simulink model "FusionMODEL_version1"  (R2018a)
settings: Solver=FixedStepAuto  StartTime=0.0  StopTime=SimulationTime  FixedStep=SamplingTime  RelTol=1e-3
undefined symbols (not defined in the file or in its folder): ACTIVATE_CAM, ACTIVATE_RAD, CAM1_detTimeStamp, CAM1_MeasNoise, CAM1_objClassID, CAM1_PX, CAM1_PY, CAM1_VX, CAM1_VY, CAM2_detTimeStamp, CAM2_MeasNoise, CAM2_objClassID, CAM2_PX, CAM2_PY, CAM2_VX, CAM2_VY, CAM3_detTimeStamp, CAM3_MeasNoise, CAM3_objClassID, CAM3_PX, CAM3_PY, CAM3_VX, CAM3_VY, CAM4_detTimeStamp, CAM4_MeasNoise, CAM4_objClassID, CAM4_PX, CAM4_PY, CAM4_VX, CAM4_VY, CAM5_detTimeStamp, CAM5_MeasNoise, CAM5_objClassID, CAM5_PX, CAM5_PY, CAM5_VX, CAM5_VY, CAM6_detTimeStamp, CAM6_MeasNoise, CAM6_objClassID, CAM6_PX, CAM6_PY, CAM6_VX, CAM6_VY, CAM7_detTimeStamp, CAM7_MeasNoise, CAM7_objClassID, CAM7_PX, CAM7_PY, CAM7_VX, CAM7_VY, CAM8_detTimeStamp, CAM8_MeasNoise, CAM8_objClassID, CAM8_PX, CAM8_PY, CAM8_VX, CAM8_VY, CAM_nMeas, CAM_TYPE ... (+151)
libraries: simulink_extras x2
(part 3 of 6)

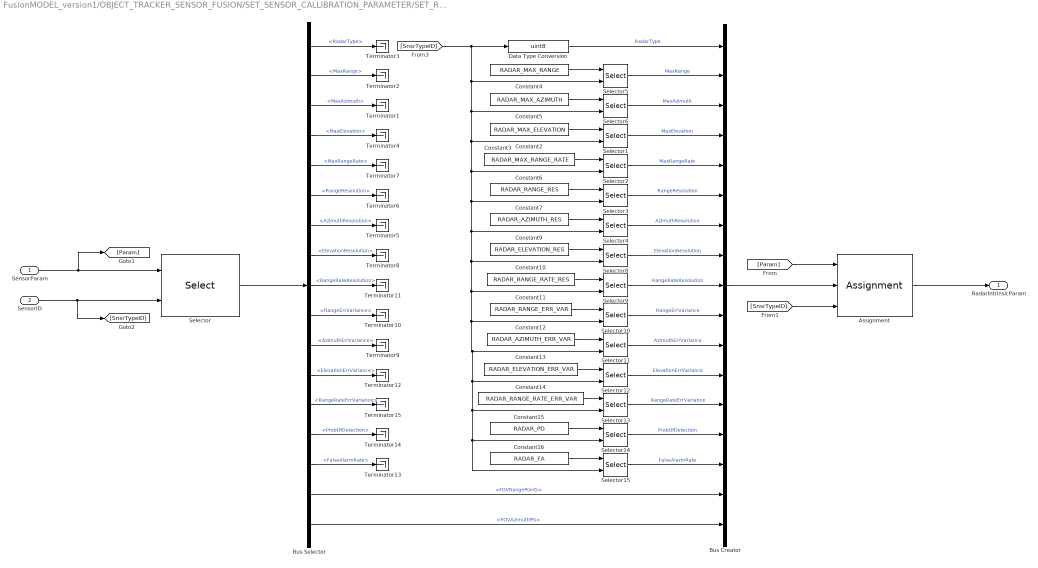
== system FusionMODEL_version1/OBJECT_TRACKER_SENSOR_FUSION/SET_SENSOR_CALLIBRATION_PARAMETER/SET_RADAR_SENSOR_PARAM/SET_RADAR_INTRINSIC_PARAM/SET_RADAR_INTRINSIC_PARAM ==
  SensorParam : Inport
  SensorID : Inport  Port=2
  Assignment : Assignment  DiagnosticForDimensions=Warning  IndexOptions=Index vector (port)  Indices=1  OutputSizes=1
  Bus Creator : BusCreator  Inputs=17  OutDataTypeStr=Bus: RadarIntrinsicParam  NonVirtualBus=on
  Bus Selector : BusSelector  OutputSignals=RadarType,MaxRange,MaxAzimuth,MaxElevation,MaxRangeRate,RangeResolution,AzimuthResolution,ElevationResolution,RangeRateResolution,RangeErrVariance,AzimuthErrVariance,ElevationErrVariance,RangeRateErrVariance,ProbOfDetection,FalseAlarmRate,FOVRangePoints,FOVAzimuthPts
  Constant10 : Constant  Value=RADAR_RANGE_RATE_RES
  Constant11 : Constant  Value=RADAR_RANGE_ERR_VAR
  Constant12 : Constant  Value=RADAR_AZIMUTH_ERR_VAR
  Constant13 : Constant  Value=RADAR_ELEVATION_ERR_VAR
  Constant14 : Constant  Value=RADAR_RANGE_RATE_ERR_VAR
  Constant15 : Constant  Value=RADAR_PD
  Constant16 : Constant  Value=RADAR_FA
  Constant2 : Constant  Value=RADAR_MAX_ELEVATION
  Constant3 : Constant  Value=RADAR_MAX_RANGE_RATE
  Constant4 : Constant  Value=RADAR_MAX_RANGE
  Constant5 : Constant  Value=RADAR_MAX_AZIMUTH
  Constant6 : Constant  Value=RADAR_RANGE_RES
  Constant7 : Constant  Value=RADAR_AZIMUTH_RES
  Constant9 : Constant  Value=RADAR_ELEVATION_RES
  Data Type Conversion : DataTypeConversion  OutDataTypeStr=uint8
  Selector{,1..6,8..15} (15 alike) : Selector  InputPortWidth=nRadarTypes  IndexOptions=Index vector (port)  Indices=[1 3]  OutputSizes=1
  Terminator{1..15} (15 alike) : Terminator
  RadarIntrinsicParam : Outport
  wires:
  Assignment/1 -> RadarIntrinsicParam/1
  SensorParam/1 -> [Param], Selector/1
  Selector/1 -> Bus Selector/1
  Bus Creator/1 -> Assignment/2
  SensorID/1 -> [SnsrTypeID], Selector/2
  [Param] -> Assignment/1
  [SnsrTypeID] -> Assignment/3
  Bus Selector/17 -> Bus Creator/17  "<FOVAzimuthPts>"
  Bus Selector/16 -> Bus Creator/16  "<FOVRangePoints>"
  Constant5/1 -> Selector6/1
  Constant4/1 -> Selector5/1
  Bus Selector/3 -> Terminator1/1  "<MaxAzimuth>"
  Bus Selector/2 -> Terminator2/1  "<MaxRange>"
  Bus Selector/1 -> Terminator3/1  "<RadarType>"
  Selector6/1 -> Bus Creator/3  "MaxAzimuth"
  Selector5/1 -> Bus Creator/2  "MaxRange"
  [SnsrTypeID] -> Selector14/2, Selector15/2, Selector13/2, Selector12/2, Selector11/2, Selector10/2, Selector9/2, Selector8/2, Selector4/2, Selector3/2, Selector2/2, Selector1/2, Selector6/2, Selector5/2, Data Type Conversion/1
  Selector1/1 -> Bus Creator/4  "MaxElevation"
  Selector2/1 -> Bus Creator/5  "MaxRangeRate"
  Selector3/1 -> Bus Creator/6  "RangeResolution"
  Selector4/1 -> Bus Creator/7  "AzimuthResolution"
  Selector8/1 -> Bus Creator/8  "ElevationResolution"
  Constant2/1 -> Selector1/1
  Constant3/1 -> Selector2/1
  Constant6/1 -> Selector3/1
  Constant7/1 -> Selector4/1
  Constant9/1 -> Selector8/1
  Selector9/1 -> Bus Creator/9  "RangeRateResolution"
  Selector10/1 -> Bus Creator/10  "RangeErrVariance"
  Selector11/1 -> Bus Creator/11  "AzimuthErrVariance"
  Selector12/1 -> Bus Creator/12  "ElevationErrVariance"
  Selector13/1 -> Bus Creator/13  "RangeRateErrVariance"
  Selector14/1 -> Bus Creator/14  "ProbOfDetection"
  Selector15/1 -> Bus Creator/15  "FalseAlarmRate"
  Constant10/1 -> Selector9/1
  Constant11/1 -> Selector10/1
  Constant12/1 -> Selector11/1
  Constant13/1 -> Selector12/1
  Constant14/1 -> Selector13/1
  Constant15/1 -> Selector14/1
  Constant16/1 -> Selector15/1
  Bus Selector/4 -> Terminator4/1  "<MaxElevation>"
  Bus Selector/7 -> Terminator5/1  "<AzimuthResolution>"
  Bus Selector/6 -> Terminator6/1  "<RangeResolution>"
  Bus Selector/8 -> Terminator8/1  "<ElevationResolution>"
  Bus Selector/5 -> Terminator7/1  "<MaxRangeRate>"
  Bus Selector/11 -> Terminator9/1  "<AzimuthErrVariance>"
  Bus Selector/14 -> Terminator14/1  "<ProbOfDetection>"
  Bus Selector/10 -> Terminator10/1  "<RangeErrVariance>"
  Bus Selector/13 -> Terminator15/1  "<RangeRateErrVariance>"
  Bus Selector/12 -> Terminator12/1  "<ElevationErrVariance>"
  Bus Selector/15 -> Terminator13/1  "<FalseAlarmRate>"
  Bus Selector/9 -> Terminator11/1  "<RangeRateResolution>"
  Data Type Conversion/1 -> Bus Creator/1  "RadarType"

== system FusionMODEL_version1/OBJECT_TRACKER_SENSOR_FUSION/SPATIAL_ALLIGNMENT/CAMERA_MEASUREMENTS_SPATIAL_ALLIGNMENT/For Iterator Subsystem/For Iterator Subsystem ==
  CameraCalibration : Inport
  nMeas : Inport  Port=2
  CameraCAN : Inport  Port=3
  CoordinateTransformation1 : Subsystem  TreatAsAtomicUnit=on
  For Iterator : ForIterator  ResetStates=reset  IterationSource=external
  SetMeasurement : Subsystem  Commented=on
  SetMeasurement1 : Subsystem
  Subsystem : Subsystem
  nValidMeas : Outport
  CameraMeasUpd : Outport  Port=2
  CameraMeasNoiseCovUpd : Outport  Port=3
  CameraMeasRefUpd : Outport  Port=4
  wires:
  nMeas/1 -> For Iterator/1
  CameraCalibration/1 -> CoordinateTransformation1/2(SensorParam)
  CameraCAN/1 -> Subsystem/1(measCAN)
  For Iterator/1 -> [CamCANidx], Subsystem/2(measIdx)
  Subsystem/4(meas_i) -> SetMeasurement1/4(CameraMeasCAN), CoordinateTransformation1/1(meas)
  Subsystem/3(nValidMeasCnt) -> nValidMeas/1
  Subsystem/2(measID) -> [measID]
  Subsystem/1(isValid) -> CoordinateTransformation1/Action
  CoordinateTransformation1/1(measUpd) -> SetMeasurement1/1(measTransformed)
  [measID] -> SetMeasurement1/2(measID)
  [CamCANidx] -> SetMeasurement1/3(CamCANidx)
  SetMeasurement1/1(CameraCTSMatUpd) -> CameraMeasUpd/1, SetMeasurement1/5(CameraMeasCTSMat)
  SetMeasurement1/2(CameraCTSNoiseCovMatUpd) -> CameraMeasNoiseCovUpd/1, SetMeasurement1/6(CameraMeasCTSNoiseMat)
  SetMeasurement1/3(CameraCTSRefUpd) -> CameraMeasRefUpd/1, SetMeasurement1/7(CameraMeasCTSRef)

== system FusionMODEL_version1/OBJECT_TRACKER_SENSOR_FUSION/SPATIAL_ALLIGNMENT/CAMERA_MEASUREMENTS_SPATIAL_ALLIGNMENT/For Iterator Subsystem/InformationExtraction ==
  CameraCallibration : Inport
  CameraID : Inport  Port=2
  C1 : Inport  Port=3
  C2 : Inport  Port=4
  C3 : Inport  Port=5
  C4 : Inport  Port=6
  C5 : Inport  Port=7
  C6 : Inport  Port=8
  C7 : Inport  Port=9
  C8 : Inport  Port=10
  StartingIndexes : Inport  Port=11
  Bus Selector : BusSelector  OutputSignals=nMeas
  Multiport Switch : MultiPortSwitch  Inputs=8
  Reshape : Reshape  OutputDimensionality=Row vector (2-D)
  Selector : Selector  NumberOfDimensions=2  InputPortWidth=3  IndexOptions=Select all,Index vector (port)  Indices=[1 3],1  OutputSizes=1,1
  Selector1 : Selector  NumberOfDimensions=2  InputPortWidth=3  IndexOptions=Select all,Index vector (port)  Indices=[1 3],1  OutputSizes=1,1
  CameraCalib : Outport
  nCameraMeas : Outport  Port=2
  CameraCANBus : Outport  Port=3
  MeasStartingIdx : Outport  Port=4
  wires:
  CameraCallibration/1 -> Selector/1
  Selector/1 -> CameraCalib/1, Bus Selector/1
  Bus Selector/1 -> nCameraMeas/1  "<nMeas>"
  CameraID/1 -> Selector1/2, Multiport Switch/1, Selector/2
  C1/1 -> Multiport Switch/2
  C2/1 -> Multiport Switch/3
  C3/1 -> Multiport Switch/4
  C4/1 -> Multiport Switch/5
  C5/1 -> Multiport Switch/6
  C6/1 -> Multiport Switch/7
  Multiport Switch/1 -> Reshape/1
  Selector1/1 -> MeasStartingIdx/1
  StartingIndexes/1 -> Selector1/1
  Reshape/1 -> CameraCANBus/1
  C7/1 -> Multiport Switch/8
  C8/1 -> Multiport Switch/9

== system FusionMODEL_version1/OBJECT_TRACKER_SENSOR_FUSION/SPATIAL_ALLIGNMENT/CAMERA_MEASUREMENTS_SPATIAL_ALLIGNMENT/For Iterator Subsystem/Subsystem ==
  nValidMeasVectorIn : Inport
  SnsrIndex : Inport  Port=2
  nValidMeas : Inport  Port=3
  CameraCTSMeas : Inport  Port=4
  CameraCTSNoiseCOV : Inport  Port=5
  CameraCTSRef : Inport  Port=6
  StartIdx : Inport  Port=7
  CTSMeasAllSensors : Inport  Port=8
  CTSNoiseCOV : Inport  Port=9
  CTSRef : Inport  Port=10
  Add : Sum
  Assignment : Assignment  NumberOfDimensions=2  DiagnosticForDimensions=Warning  IndexOptions=Assign all,Index vector (port)  Indices=1,1  OutputSizes=1,1
  Assignment1 : Assignment  NumberOfDimensions=2  DiagnosticForDimensions=Warning  IndexOptions=Assign all,Starting index (port)  Indices=1,1  OutputSizes=1,1
  Assignment2 : Assignment  NumberOfDimensions=3  DiagnosticForDimensions=Warning  IndexOptions=Assign all,Assign all,Starting index (port)  Indices=1,1,1  OutputSizes=1,1,1
  Assignment3 : Assignment  NumberOfDimensions=2  DiagnosticForDimensions=Warning  IndexOptions=Assign all,Starting index (port)  Indices=1,1  OutputSizes=1,1
  Constant2 : Constant  Value=int32(1)
  Data Type Conversion : DataTypeConversion  OutDataTypeStr=uint16
  Reshape : Reshape  OutputDimensionality=Row vector (2-D)
  Unit Delay : UnitDelay  InitialCondition=single(zeros(2, 1600))  SampleTime=-1
  Unit Delay1 : UnitDelay  InitialCondition=uint16(zeros(1,8))  SampleTime=-1
  Unit Delay2 : UnitDelay  InitialCondition=single(zeros(2, 2, 1600))  SampleTime=-1
  Unit Delay3 : UnitDelay  InitialCondition=uint16(zeros(2, 1600))  SampleTime=-1
  nValidMeasVector : Outport
  CTSMat : Outport  Port=2
  CTSMatNoiseCOV : Outport  Port=3
  CTSMatRef : Outport  Port=4
  wires:
  nValidMeas/1 -> Data Type Conversion/1
  SnsrIndex/1 -> Assignment/3
  Assignment/1 -> nValidMeasVector/1
  Unit Delay1/1 -> Reshape/1
  CTSMeasAllSensors/1 -> Unit Delay/1
  CameraCTSMeas/1 -> Assignment1/2
  Assignment1/1 -> CTSMat/1
  StartIdx/1 -> Add/1
  Constant2/1 -> Add/2
  Data Type Conversion/1 -> Assignment/2
  Reshape/1 -> Assignment/1
  nValidMeasVectorIn/1 -> Unit Delay1/1
  Unit Delay/1 -> Assignment1/1
  Unit Delay2/1 -> Assignment2/1
  CameraCTSNoiseCOV/1 -> Assignment2/2
  Add/1 -> Assignment3/3, Assignment2/3, Assignment1/3
  Assignment2/1 -> CTSMatNoiseCOV/1
  Assignment3/1 -> CTSMatRef/1
  CameraCTSRef/1 -> Assignment3/2
  Unit Delay3/1 -> Assignment3/1
  CTSNoiseCOV/1 -> Unit Delay2/1
  CTSRef/1 -> Unit Delay3/1

== system FusionMODEL_version1/OBJECT_TRACKER_SENSOR_FUSION/SPATIAL_ALLIGNMENT/CAMERA_MEASUREMENTS_SPATIAL_ALLIGNMENT/StartingIndexes1/CallibrationInfoExtractor ==
  SnsrCallib : Inport
  Bus Selector{,1..7} (8 alike) : BusSelector  OutputSignals=nMeas
  Selector : Selector  InputPortWidth=nCameras  IndexOptions=Index vector (dialog)  Indices=1  OutputSizes=1
  Selector1 : Selector  InputPortWidth=nCameras  IndexOptions=Index vector (dialog)  Indices=2  OutputSizes=1
  Selector2 : Selector  InputPortWidth=nCameras  IndexOptions=Index vector (dialog)  Indices=3  OutputSizes=1
  Selector3 : Selector  InputPortWidth=nCameras  IndexOptions=Index vector (dialog)  Indices=4  OutputSizes=1
  Selector4 : Selector  InputPortWidth=nCameras  IndexOptions=Index vector (dialog)  Indices=5  OutputSizes=1
  Selector5 : Selector  InputPortWidth=nCameras  IndexOptions=Index vector (dialog)  Indices=7  OutputSizes=1
  Selector6 : Selector  InputPortWidth=nCameras  IndexOptions=Index vector (dialog)  Indices=6  OutputSizes=1
  Selector7 : Selector  InputPortWidth=nCameras  IndexOptions=Index vector (dialog)  Indices=8  OutputSizes=1
  Terminator : Terminator
  C1nMeas : Outport
  C2nMeas : Outport  Port=2
  C3nMeas : Outport  Port=3
  C4nMeas : Outport  Port=4
  C5nMeas : Outport  Port=5
  C6nMeas : Outport  Port=6
  C7nMeas : Outport  Port=7
  wires:
  Bus Selector4/1 -> C5nMeas/1  "<nMeas>"
  Selector4/1 -> Bus Selector4/1
  Bus Selector1/1 -> C2nMeas/1  "<nMeas>"
  Selector1/1 -> Bus Selector1/1
  Selector2/1 -> Bus Selector2/1
  Bus Selector2/1 -> C3nMeas/1  "<nMeas>"
  Selector6/1 -> Bus Selector5/1
  Selector/1 -> Bus Selector/1
  Selector3/1 -> Bus Selector3/1
  Bus Selector3/1 -> C4nMeas/1  "<nMeas>"
  Bus Selector/1 -> C1nMeas/1  "<nMeas>"
  Bus Selector5/1 -> C6nMeas/1  "<nMeas>"
  Selector5/1 -> Bus Selector6/1
  Bus Selector6/1 -> C7nMeas/1  "<nMeas>"
  Bus Selector7/1 -> Terminator/1  "<nMeas>"
  Selector7/1 -> Bus Selector7/1
  SnsrCallib/1 -> Selector7/1, Selector5/1, Selector6/1, Selector4/1, Selector3/1, Selector2/1, Selector1/1, Selector/1

== system FusionMODEL_version1/OBJECT_TRACKER_SENSOR_FUSION/SPATIAL_ALLIGNMENT/CAMERA_MEASUREMENTS_SPATIAL_ALLIGNMENT/StartingIndexes1/Subsystem ==
  C1nMeas : Inport
  C2nMeas : Inport  Port=2
  C3nMeas : Inport  Port=3
  C4nMeas : Inport  Port=4
  C5nMeas : Inport  Port=5
  C6nMeas : Inport  Port=6
  C7nMeas : Inport  Port=7
  Add{,1..5} (6 alike) : Sum
  Constant : Constant  Value=int32(0)
  Data Type Conversion{,1..6} (7 alike) : DataTypeConversion  OutDataTypeStr=int32
  Mux : Mux  Inputs=8
  Reshape : Reshape  OutputDimensionality=Row vector (2-D)
  StartingIndexes : Outport
  wires:
  [C1] -> Mux/1
  Add/1 -> [C3], Add1/1
  Add1/1 -> [C4], Add2/1
  Data Type Conversion3/1 -> Add2/2
  [C4] -> Mux/4
  [C2] -> Mux/2
  Add3/1 -> Add4/1, [C6]
  Constant/1 -> [C1]
  Add2/1 -> [C5], Add3/1
  [C5] -> Mux/5
  [C6] -> Mux/6
  C5nMeas/1 -> Data Type Conversion4/1
  Data Type Conversion/1 -> [C2], Add/1
  [C3] -> Mux/3
  Data Type Conversion1/1 -> Add/2
  Data Type Conversion2/1 -> Add1/2
  Data Type Conversion4/1 -> Add3/2
  C3nMeas/1 -> Data Type Conversion2/1
  C1nMeas/1 -> Data Type Conversion/1
  C2nMeas/1 -> Data Type Conversion1/1
  Mux/1 -> Reshape/1
  C4nMeas/1 -> Data Type Conversion3/1
  Reshape/1 -> StartingIndexes/1
  C6nMeas/1 -> Data Type Conversion5/1
  C7nMeas/1 -> Data Type Conversion6/1
  Data Type Conversion5/1 -> Add4/2
  Data Type Conversion6/1 -> Add5/2
  Add4/1 -> [C7], Add5/1
  Add5/1 -> [C8]
  [C7] -> Mux/7
  [C8] -> Mux/8

== system FusionMODEL_version1/OBJECT_TRACKER_SENSOR_FUSION/SPATIAL_ALLIGNMENT/RADAR_MEASUREMENTS_SPATIAL_ALLIGNMENT/RADAR_MEASUREMENTS_SPATIAL_ALLIGNMENT/COORDINATE_TRANSFORMATION ==
  RadarCalibration : Inport
  nMeas : Inport  Port=2
  RadarCAN : Inport  Port=3
  COORDINATE_TRANSFORMATION : Subsystem  TreatAsAtomicUnit=on
  GET_DATA : Subsystem
  MEASUREMENT_LOOP : ForIterator  ResetStates=reset  IterationSource=external
  SET_DATA : Subsystem
  nValidMeas : Outport
  RadarMeasUpd : Outport  Port=2
  RadarMeasNoiseCovUpd : Outport  Port=3
  RadarMeasRefUpd : Outport  Port=4
  wires:
  nMeas/1 -> MEASUREMENT_LOOP/1
  RadarCalibration/1 -> COORDINATE_TRANSFORMATION/2(SensorParam)
  RadarCAN/1 -> GET_DATA/1(measCAN)
  MEASUREMENT_LOOP/1 -> [RadCANidx], GET_DATA/2(measIdx)
  GET_DATA/4(meas_i) -> SET_DATA/4(RadarMeasCAN), COORDINATE_TRANSFORMATION/1(meas)
  GET_DATA/3(nValidMeasCnt) -> nValidMeas/1
  GET_DATA/2(measID) -> [measID]
  COORDINATE_TRANSFORMATION/1(measUpd) -> SET_DATA/1(measTransformed)
  [measID] -> SET_DATA/2(measID)
  [RadCANidx] -> SET_DATA/3(RadCANidx)
  SET_DATA/1(RadarCTSMatUpd) -> RadarMeasUpd/1, SET_DATA/5(RadarMeasCTSMat)
  GET_DATA/1(isValid) -> COORDINATE_TRANSFORMATION/Action
  SET_DATA/3(RadarCTSRefUpd) -> RadarMeasRefUpd/1, SET_DATA/7(RadarMeasCTSRef)
  SET_DATA/2(RadarCTSNoiseCovMatUpd) -> RadarMeasNoiseCovUpd/1, SET_DATA/6(RadarMeasCTSNoiseMat)

== system FusionMODEL_version1/OBJECT_TRACKER_SENSOR_FUSION/SPATIAL_ALLIGNMENT/RADAR_MEASUREMENTS_SPATIAL_ALLIGNMENT/RADAR_MEASUREMENTS_SPATIAL_ALLIGNMENT/GET_DATA ==
  RadarCallibration : Inport
  RadarID : Inport  Port=2
  R1 : Inport  Port=3
  R2 : Inport  Port=4
  R3 : Inport  Port=5
  R4 : Inport  Port=6
  R5 : Inport  Port=7
  R6 : Inport  Port=8
  StartingIndexes : Inport  Port=9
  Bus Selector : BusSelector  OutputSignals=nMeas
  Multiport Switch : MultiPortSwitch  Inputs=6
  Reshape : Reshape  OutputDimensionality=Row vector (2-D)
  Selector : Selector  NumberOfDimensions=2  InputPortWidth=3  IndexOptions=Select all,Index vector (port)  Indices=[1 3],1  OutputSizes=1,1
  Selector1 : Selector  NumberOfDimensions=2  InputPortWidth=3  IndexOptions=Select all,Index vector (port)  Indices=[1 3],1  OutputSizes=1,1
  RadarCalib : Outport
  nRadarMeas : Outport  Port=2
  RadarCANBus : Outport  Port=3
  MeasStartingIdx : Outport  Port=4
  wires:
  RadarCallibration/1 -> Selector/1
  Selector/1 -> RadarCalib/1, Bus Selector/1
  Bus Selector/1 -> nRadarMeas/1  "<nMeas>"
  RadarID/1 -> Selector1/2, Selector/2, Multiport Switch/1
  R1/1 -> Multiport Switch/2
  R2/1 -> Multiport Switch/3
  R3/1 -> Multiport Switch/4
  R4/1 -> Multiport Switch/5
  R5/1 -> Multiport Switch/6
  R6/1 -> Multiport Switch/7
  Multiport Switch/1 -> Reshape/1
  Selector1/1 -> MeasStartingIdx/1
  StartingIndexes/1 -> Selector1/1
  Reshape/1 -> RadarCANBus/1

== system FusionMODEL_version1/OBJECT_TRACKER_SENSOR_FUSION/SPATIAL_ALLIGNMENT/RADAR_MEASUREMENTS_SPATIAL_ALLIGNMENT/RADAR_MEASUREMENTS_SPATIAL_ALLIGNMENT/SET_DATA ==
  nValidMeasVectorIn : Inport
  SnsrIndex : Inport  Port=2
  nValidMeas : Inport  Port=3
  RadarCTSMeas : Inport  Port=4
  RadarCTSNoiseCOV : Inport  Port=5
  RadarCTSRef : Inport  Port=6
  StartIdx : Inport  Port=7
  CTSMeasAllSensors : Inport  Port=8
  CTSNoiseCOV : Inport  Port=9
  CTSRef : Inport  Port=10
  Add : Sum
  Assignment : Assignment  NumberOfDimensions=2  DiagnosticForDimensions=Warning  IndexOptions=Assign all,Index vector (port)  Indices=1,1  OutputSizes=1,1
  Assignment1 : Assignment  NumberOfDimensions=2  DiagnosticForDimensions=Warning  IndexOptions=Assign all,Starting index (port)  Indices=1,1  OutputSizes=1,1
  Assignment2 : Assignment  NumberOfDimensions=3  DiagnosticForDimensions=Warning  IndexOptions=Assign all,Assign all,Starting index (port)  Indices=1,1,1  OutputSizes=1,1,1
  Assignment3 : Assignment  NumberOfDimensions=2  DiagnosticForDimensions=Warning  IndexOptions=Assign all,Starting index (port)  Indices=1,1  OutputSizes=1,1
  Constant2 : Constant  Value=int32(1)
  Data Type Conversion : DataTypeConversion  OutDataTypeStr=uint16
  Reshape : Reshape  OutputDimensionality=Row vector (2-D)
  Unit Delay : UnitDelay  InitialCondition=single(zeros(2, 1200))  SampleTime=-1
  Unit Delay1 : UnitDelay  InitialCondition=uint16(zeros(1,6))  SampleTime=-1
  Unit Delay2 : UnitDelay  InitialCondition=single(zeros(2, 2, 1200))  SampleTime=-1
  Unit Delay3 : UnitDelay  InitialCondition=uint16(zeros(2, 1200))  SampleTime=-1
  nValidMeasVector : Outport
  CTSMat : Outport  Port=2
  CTSMatNoiseCOV : Outport  Port=3
  CTSMatRef : Outport  Port=4
  wires:
  nValidMeas/1 -> Data Type Conversion/1
  SnsrIndex/1 -> Assignment/3
  Assignment/1 -> nValidMeasVector/1
  Unit Delay1/1 -> Reshape/1
  CTSMeasAllSensors/1 -> Unit Delay/1
  RadarCTSMeas/1 -> Assignment1/2
  Assignment1/1 -> CTSMat/1
  StartIdx/1 -> Add/1
  Constant2/1 -> Add/2
  Data Type Conversion/1 -> Assignment/2
  Reshape/1 -> Assignment/1
  nValidMeasVectorIn/1 -> Unit Delay1/1
  Unit Delay/1 -> Assignment1/1
  Unit Delay2/1 -> Assignment2/1
  RadarCTSNoiseCOV/1 -> Assignment2/2
  Add/1 -> Assignment3/3, Assignment2/3, Assignment1/3
  Assignment2/1 -> CTSMatNoiseCOV/1
  Assignment3/1 -> CTSMatRef/1
  RadarCTSRef/1 -> Assignment3/2
  Unit Delay3/1 -> Assignment3/1
  CTSNoiseCOV/1 -> Unit Delay2/1
  CTSRef/1 -> Unit Delay3/1

== system FusionMODEL_version1/OBJECT_TRACKER_SENSOR_FUSION/SPATIAL_ALLIGNMENT/RADAR_MEASUREMENTS_SPATIAL_ALLIGNMENT/StartingIndexes1/CallibrationInfoExtractor ==
  SnsrCallib : Inport
  Bus Selector{,1..5} (6 alike) : BusSelector  OutputSignals=nMeas
  Selector : Selector  InputPortWidth=nRadars  IndexOptions=Index vector (dialog)  Indices=1  OutputSizes=1
  Selector1 : Selector  InputPortWidth=nRadars  IndexOptions=Index vector (dialog)  Indices=2  OutputSizes=1
  Selector2 : Selector  InputPortWidth=nRadars  IndexOptions=Index vector (dialog)  Indices=3  OutputSizes=1
  Selector3 : Selector  InputPortWidth=nRadars  IndexOptions=Index vector (dialog)  Indices=4  OutputSizes=1
  Selector4 : Selector  InputPortWidth=nRadars  IndexOptions=Index vector (dialog)  Indices=5  OutputSizes=1
  Selector5 : Selector  InputPortWidth=nRadars  IndexOptions=Index vector (dialog)  Indices=6  OutputSizes=1
  Terminator : Terminator
  R1nMeas : Outport
  R2nMeas : Outport  Port=2
  R3nMeas : Outport  Port=3
  R4nMeas : Outport  Port=4
  R5nMeas : Outport  Port=5
  wires:
  Bus Selector4/1 -> R5nMeas/1  "<nMeas>"
  Selector4/1 -> Bus Selector4/1
  SnsrCallib/1 -> Selector1/1, Selector2/1, Selector3/1, Selector5/1, Selector4/1, Selector/1
  Bus Selector1/1 -> R2nMeas/1  "<nMeas>"
  Selector1/1 -> Bus Selector1/1
  Selector2/1 -> Bus Selector2/1
  Bus Selector2/1 -> R3nMeas/1  "<nMeas>"
  Selector5/1 -> Bus Selector5/1
  Selector/1 -> Bus Selector/1
  Selector3/1 -> Bus Selector3/1
  Bus Selector5/1 -> Terminator/1  "<nMeas>"
  Bus Selector3/1 -> R4nMeas/1  "<nMeas>"
  Bus Selector/1 -> R1nMeas/1  "<nMeas>"

== system FusionMODEL_version1/OBJECT_TRACKER_SENSOR_FUSION/SPATIAL_ALLIGNMENT/RADAR_MEASUREMENTS_SPATIAL_ALLIGNMENT/StartingIndexes1/Subsystem ==
  R1nMeas : Inport
  R2nMeas : Inport  Port=2
  R3nMeas : Inport  Port=3
  R4nMeas : Inport  Port=4
  R5nMeas : Inport  Port=5
  Add{,1..3} (4 alike) : Sum
  Constant : Constant  Value=int32(0)
  Data Type Conversion{,1..4} (5 alike) : DataTypeConversion  OutDataTypeStr=int32
  Mux : Mux  Inputs=6
  Reshape : Reshape  OutputDimensionality=Row vector (2-D)
  StartingIndexes : Outport
  wires:
  [R1] -> Mux/1
  Add/1 -> [R3], Add1/1
  Add1/1 -> [R4], Add2/1
  Data Type Conversion3/1 -> Add2/2
  [R4] -> Mux/4
  [R2] -> Mux/2
  Add3/1 -> [R6]
  Constant/1 -> [R1]
  Add2/1 -> [R5], Add3/1
  [R5] -> Mux/5
  [R6] -> Mux/6
  R5nMeas/1 -> Data Type Conversion4/1
  Data Type Conversion/1 -> [R2], Add/1
  [R3] -> Mux/3
  Data Type Conversion1/1 -> Add/2
  Data Type Conversion2/1 -> Add1/2
  Data Type Conversion4/1 -> Add3/2
  R3nMeas/1 -> Data Type Conversion2/1
  R1nMeas/1 -> Data Type Conversion/1
  R2nMeas/1 -> Data Type Conversion1/1
  Mux/1 -> Reshape/1
  R4nMeas/1 -> Data Type Conversion3/1
  Reshape/1 -> StartingIndexes/1

== system FusionMODEL_version1/SENSOR_MEASUREMENTS/RADAR_CAMERA_EGO_SENSOR_INTERFACE/CameraSensors/Camera1/CHECK_IF_DATA_IS_VALID ==
  idx : Inport
  px : Inport  Port=2
  py : Inport  Port=3
  vx : Inport  Port=4
  vy : Inport  Port=5
  Abs{,1..3} (4 alike) : Abs
  Add : Sum  Inputs=++++
  Constant : Constant  Value=uint16(0)
  Data Type Conversion : DataTypeConversion  OutDataTypeStr=uint16
  Switch : Switch  Threshold=0.0001
  ID : Outport
  wires:
  Add/1 -> Switch/2
  Abs2/1 -> Add/3
  Constant/1 -> Switch/3
  Abs/1 -> Add/1
  px/1 -> Abs/1
  Abs3/1 -> Add/4
  Abs1/1 -> Add/2
  vy/1 -> Abs3/1
  py/1 -> Abs1/1
  vx/1 -> Abs2/1
  idx/1 -> Data Type Conversion/1
  Switch/1 -> ID/1
  Data Type Conversion/1 -> Switch/1

== system FusionMODEL_version1/SENSOR_MEASUREMENTS/RADAR_CAMERA_EGO_SENSOR_INTERFACE/CameraSensors/Camera1/GET_DATA ==
  idx : Inport
  time : Inport  Port=2
  Constant : Constant  Value=CAM1_PX
  Constant1 : Constant  Value=CAM1_PY
  Constant2 : Constant  Value=CAM1_VX
  Constant3 : Constant  Value=CAM1_VY
  Constant4 : Constant  Value=CAM1_objClassID
  Constant5 : Constant  Value=CAM1_MeasNoise
  Constant6 : Constant  Value=CAM1_detTimeStamp
  Data Type Conversion : DataTypeConversion  OutDataTypeStr=int16
  MeasNoise : Selector  NumberOfDimensions=4  InputPortWidth=3  IndexOptions=Index vector (port),Select all,Select all,Index vector (port)  Indices=[1 3],1,1,1  OutputSizes=1,1,1,1
  ObjectClass : Selector  NumberOfDimensions=2  InputPortWidth=3  IndexOptions=Index vector (port),Index vector (port)  Indices=[1 3],1  OutputSizes=1,1
  PosX : Selector  NumberOfDimensions=2  InputPortWidth=3  IndexOptions=Index vector (port),Index vector (port)  Indices=[1 3],1  OutputSizes=1,1
  PosY : Selector  NumberOfDimensions=2  InputPortWidth=3  IndexOptions=Index vector (port),Index vector (port)  Indices=[1 3],1  OutputSizes=1,1
  Reshape : Reshape  OutputDimensionality=Customize  OutputDimensions=[4,4]
  VelX : Selector  NumberOfDimensions=2  InputPortWidth=3  IndexOptions=Index vector (port),Index vector (port)  Indices=[1 3],1  OutputSizes=1,1
  VelY : Selector  NumberOfDimensions=2  InputPortWidth=3  IndexOptions=Index vector (port),Index vector (port)  Indices=[1 3],1  OutputSizes=1,1
  timeStamp : Selector  NumberOfDimensions=2  InputPortWidth=3  IndexOptions=Select all,Index vector (port)  Indices=[1 3],1  OutputSizes=1,1
  PX : Outport
  PY : Outport  Port=2
  VX : Outport  Port=3
  VY : Outport  Port=4
  OBJ_TYPE : Outport  Port=5
  NOISE_COV : Outport  Port=6
  measCaptureTime : Outport  Port=7
  wires:
  Constant3/1 -> VelY/1
  Constant2/1 -> VelX/1
  VelY/1 -> VY/1
  Constant/1 -> PosX/1
  idx/1 -> MeasNoise/3, ObjectClass/3, VelY/3, VelX/3, PosY/3, PosX/3
  Constant1/1 -> PosY/1
  VelX/1 -> VX/1
  PosX/1 -> PX/1
  PosY/1 -> PY/1
  time/1 -> timeStamp/2, MeasNoise/2, ObjectClass/2, VelY/2, VelX/2, PosY/2, PosX/2
  Constant4/1 -> ObjectClass/1
  ObjectClass/1 -> Data Type Conversion/1
  Constant5/1 -> MeasNoise/1
  Constant6/1 -> timeStamp/1
  MeasNoise/1 -> Reshape/1
  timeStamp/1 -> measCaptureTime/1
  Reshape/1 -> NOISE_COV/1
  Data Type Conversion/1 -> OBJ_TYPE/1

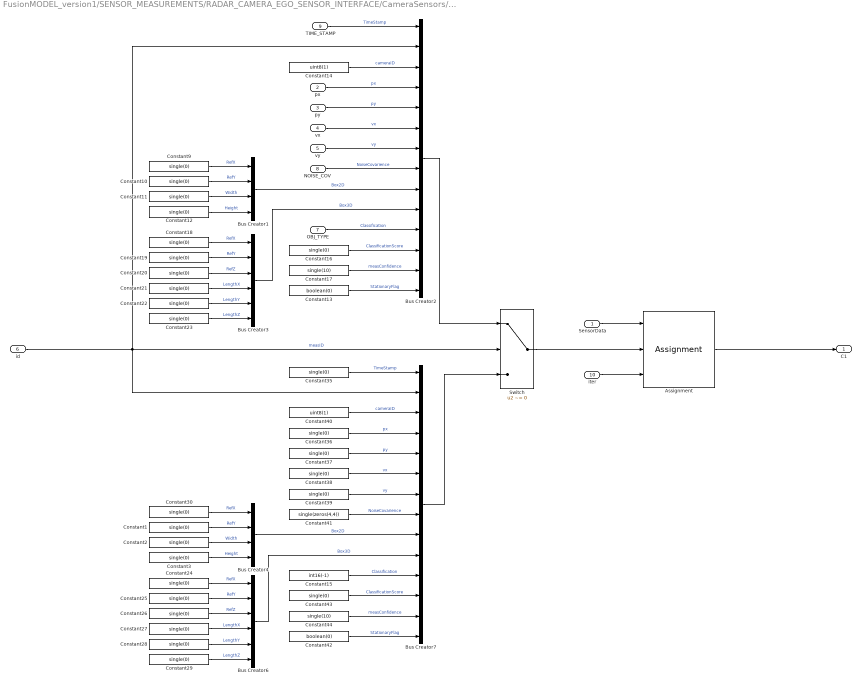
== system FusionMODEL_version1/SENSOR_MEASUREMENTS/RADAR_CAMERA_EGO_SENSOR_INTERFACE/CameraSensors/Camera1/SET_DATA ==
  SensorData : Inport
  px : Inport  Port=2
  py : Inport  Port=3
  vx : Inport  Port=4
  vy : Inport  Port=5
  id : Inport  Port=6
  OBJ_TYPE : Inport  Port=7
  NOISE_COV : Inport  Port=8
  TIME_STAMP : Inport  Port=9
  iter : Inport  Port=10
  Assignment : Assignment  DiagnosticForDimensions=Warning  IndexOptions=Index vector (port)  Indices=1  OutputSizes=1
  Bus Creator1 : BusCreator  Inputs=4  OutDataTypeStr=Bus: BoxParam2D  NonVirtualBus=on
  Bus Creator2 : BusCreator  Inputs=14  OutDataTypeStr=Bus: CameraMeasParam  NonVirtualBus=on
  Bus Creator3 : BusCreator  Inputs=6  OutDataTypeStr=Bus: BoxParam3D  NonVirtualBus=on
  Bus Creator4 : BusCreator  Inputs=4  OutDataTypeStr=Bus: BoxParam2D  NonVirtualBus=on
  Bus Creator6 : BusCreator  Inputs=6  OutDataTypeStr=Bus: BoxParam3D  NonVirtualBus=on
  Bus Creator7 : BusCreator  Inputs=14  OutDataTypeStr=Bus: CameraMeasParam  NonVirtualBus=on
  Constant{1..3,9..12,16,18..30,35..39,43} (27 alike) : Constant  Value=single(0)
  Constant13 : Constant  Value=boolean(0)
  Constant14 : Constant  Value=uint8(1)
  Constant15 : Constant  Value=int16(-1)
  Constant17 : Constant  Value=single(10)
  Constant40 : Constant  Value=uint8(1)
  Constant41 : Constant  Value=single(zeros(4,4))
  Constant42 : Constant  Value=boolean(0)
  Constant44 : Constant  Value=single(10)
  Switch : Switch  Criteria=u2 ~= 0
  C1 : Outport
  wires:
  Bus Creator4/1 -> Bus Creator7/9  "Box2D"
  Bus Creator1/1 -> Bus Creator2/9  "Box2D"
  Bus Creator7/1 -> Switch/3
  Constant3/1 -> Bus Creator4/4  "Height"
  Constant44/1 -> Bus Creator7/13  "measConfidence"
  Constant19/1 -> Bus Creator3/2  "RefY"
  id/1 -> Bus Creator7/2, Bus Creator2/2, Switch/2  "measID"
  Bus Creator2/1 -> Switch/1
  Constant2/1 -> Bus Creator4/3  "Width"
  Constant12/1 -> Bus Creator1/4  "Height"
  Constant43/1 -> Bus Creator7/12  "ClassificationScore"
  Constant41/1 -> Bus Creator7/8  "NoiseCovarience"
  Constant20/1 -> Bus Creator3/3  "RefZ"
  Constant37/1 -> Bus Creator7/5  "py"
  Constant23/1 -> Bus Creator3/6  "LengthZ"
  Constant11/1 -> Bus Creator1/3  "Width"
  Constant18/1 -> Bus Creator3/1  "RefX"
  Constant9/1 -> Bus Creator1/1  "RefX"
  Constant27/1 -> Bus Creator6/4  "LengthX"
  Bus Creator3/1 -> Bus Creator2/10  "Box3D"
  Constant17/1 -> Bus Creator2/13  "measConfidence"
  py/1 -> Bus Creator2/5  "py"
  Constant36/1 -> Bus Creator7/4  "px"
  Constant16/1 -> Bus Creator2/12  "ClassificationScore"
  Constant42/1 -> Bus Creator7/14  "StationaryFlag"
  SensorData/1 -> Assignment/1
  px/1 -> Bus Creator2/4  "px"
  Constant39/1 -> Bus Creator7/7  "vy"
  Constant35/1 -> Bus Creator7/1  "TimeStamp"
  Constant38/1 -> Bus Creator7/6  "vx"
  TIME_STAMP/1 -> Bus Creator2/1  "TimeStamp"
  Switch/1 -> Assignment/2
  iter/1 -> Assignment/3
  Bus Creator6/1 -> Bus Creator7/10  "Box3D"
  Constant10/1 -> Bus Creator1/2  "RefY"
  NOISE_COV/1 -> Bus Creator2/8  "NoiseCovarience"
  Constant21/1 -> Bus Creator3/4  "LengthX"
  Constant1/1 -> Bus Creator4/2  "RefY"
  Constant25/1 -> Bus Creator6/2  "RefY"
  Constant26/1 -> Bus Creator6/3  "RefZ"
  Constant29/1 -> Bus Creator6/6  "LengthZ"
  Constant30/1 -> Bus Creator4/1  "RefX"
  vx/1 -> Bus Creator2/6  "vx"
  Constant13/1 -> Bus Creator2/14  "StationaryFlag"
  Constant22/1 -> Bus Creator3/5  "LengthY"
  Constant24/1 -> Bus Creator6/1  "RefX"
  Constant40/1 -> Bus Creator7/3  "cameraID"
  Constant28/1 -> Bus Creator6/5  "LengthY"
  Assignment/1 -> C1/1
  Constant15/1 -> Bus Creator7/11  "Classification"
  Constant14/1 -> Bus Creator2/3  "cameraID"
  vy/1 -> Bus Creator2/7  "vy"
  OBJ_TYPE/1 -> Bus Creator2/11  "Classification"

== system FusionMODEL_version1/SENSOR_MEASUREMENTS/RADAR_CAMERA_EGO_SENSOR_INTERFACE/CameraSensors/Camera2/ExtractMeasParam1 ==
  idx : Inport
  time : Inport  Port=2
  Constant : Constant  Value=CAM2_PX
  Constant1 : Constant  Value=CAM2_PY
  Constant2 : Constant  Value=CAM2_VX
  Constant3 : Constant  Value=CAM2_VY
  Constant4 : Constant  Value=CAM2_objClassID
  Constant5 : Constant  Value=CAM2_MeasNoise
  Constant6 : Constant  Value=CAM2_detTimeStamp
  Data Type Conversion : DataTypeConversion  OutDataTypeStr=int16
  MeasNoise : Selector  NumberOfDimensions=4  InputPortWidth=3  IndexOptions=Index vector (port),Select all,Select all,Index vector (port)  Indices=[1 3],1,1,1  OutputSizes=1,1,1,1
  PosX : Selector  NumberOfDimensions=2  InputPortWidth=3  IndexOptions=Index vector (port),Index vector (port)  Indices=[1 3],1  OutputSizes=1,1
  PosY : Selector  NumberOfDimensions=2  InputPortWidth=3  IndexOptions=Index vector (port),Index vector (port)  Indices=[1 3],1  OutputSizes=1,1
  Reshape : Reshape  OutputDimensionality=Customize  OutputDimensions=[4,4]
  VelX : Selector  NumberOfDimensions=2  InputPortWidth=3  IndexOptions=Index vector (port),Index vector (port)  Indices=[1 3],1  OutputSizes=1,1
  VelY : Selector  NumberOfDimensions=2  InputPortWidth=3  IndexOptions=Index vector (port),Index vector (port)  Indices=[1 3],1  OutputSizes=1,1
  snr : Selector  NumberOfDimensions=2  InputPortWidth=3  IndexOptions=Index vector (port),Index vector (port)  Indices=[1 3],1  OutputSizes=1,1
  timeStamp : Selector  NumberOfDimensions=2  InputPortWidth=3  IndexOptions=Select all,Index vector (port)  Indices=[1 3],1  OutputSizes=1,1
  PX : Outport
  PY : Outport  Port=2
  VX : Outport  Port=3
  VY : Outport  Port=4
  OBJ_TYPE : Outport  Port=5
  NOISE_COV : Outport  Port=6
  measCaptureTime : Outport  Port=7
  wires:
  Constant3/1 -> VelY/1
  Constant2/1 -> VelX/1
  VelY/1 -> VY/1
  Constant/1 -> PosX/1
  idx/1 -> MeasNoise/3, snr/3, VelY/3, VelX/3, PosY/3, PosX/3
  Constant1/1 -> PosY/1
  VelX/1 -> VX/1
  PosX/1 -> PX/1
  PosY/1 -> PY/1
  time/1 -> timeStamp/2, MeasNoise/2, snr/2, VelY/2, VelX/2, PosY/2, PosX/2
  Constant4/1 -> snr/1
  snr/1 -> Data Type Conversion/1
  Constant5/1 -> MeasNoise/1
  Constant6/1 -> timeStamp/1
  MeasNoise/1 -> Reshape/1
  timeStamp/1 -> measCaptureTime/1
  Reshape/1 -> NOISE_COV/1
  Data Type Conversion/1 -> OBJ_TYPE/1

== system FusionMODEL_version1/SENSOR_MEASUREMENTS/RADAR_CAMERA_EGO_SENSOR_INTERFACE/CameraSensors/Camera2/IsValid2 ==
  idx : Inport
  px : Inport  Port=2
  py : Inport  Port=3
  vx : Inport  Port=4
  vy : Inport  Port=5
  Abs{,1..3} (4 alike) : Abs
  Add : Sum  Inputs=++++
  Constant : Constant  Value=uint16(0)
  Data Type Conversion : DataTypeConversion  OutDataTypeStr=uint16
  Switch : Switch  Threshold=0.0001
  ID : Outport
  wires:
  Add/1 -> Switch/2
  Abs2/1 -> Add/3
  Constant/1 -> Switch/3
  Abs/1 -> Add/1
  px/1 -> Abs/1
  Abs3/1 -> Add/4
  Abs1/1 -> Add/2
  vy/1 -> Abs3/1
  py/1 -> Abs1/1
  vx/1 -> Abs2/1
  idx/1 -> Data Type Conversion/1
  Switch/1 -> ID/1
  Data Type Conversion/1 -> Switch/1

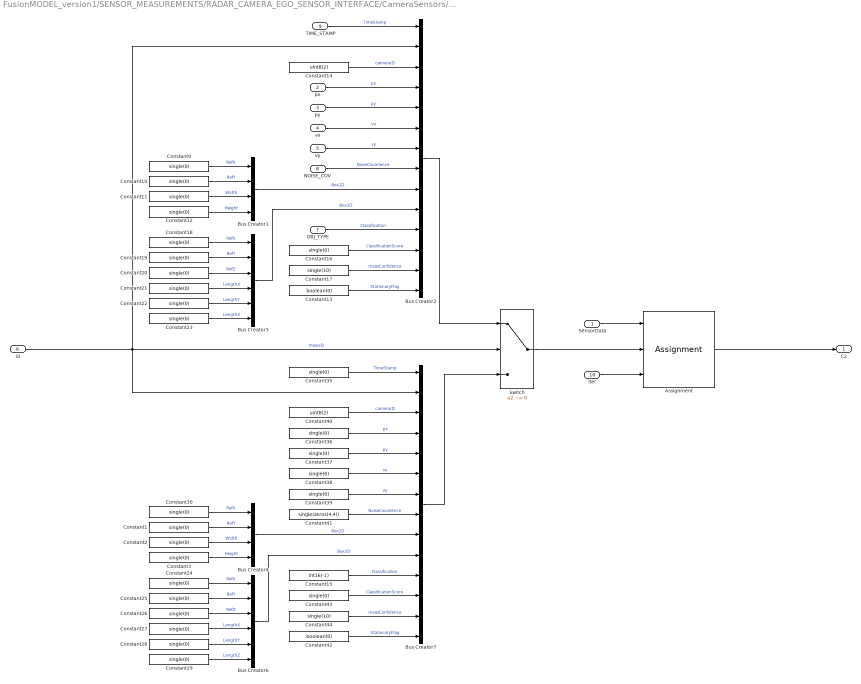
== system FusionMODEL_version1/SENSOR_MEASUREMENTS/RADAR_CAMERA_EGO_SENSOR_INTERFACE/CameraSensors/Camera2/Subsystem1 ==
  SensorData : Inport
  px : Inport  Port=2
  py : Inport  Port=3
  vx : Inport  Port=4
  vy : Inport  Port=5
  id : Inport  Port=6
  OBJ_TYPE : Inport  Port=7
  NOISE_COV : Inport  Port=8
  TIME_STAMP : Inport  Port=9
  iter : Inport  Port=10
  Assignment : Assignment  DiagnosticForDimensions=Warning  IndexOptions=Index vector (port)  Indices=1  OutputSizes=1
  Bus Creator1 : BusCreator  Inputs=4  OutDataTypeStr=Bus: BoxParam2D  NonVirtualBus=on
  Bus Creator2 : BusCreator  Inputs=14  OutDataTypeStr=Bus: CameraMeasParam  NonVirtualBus=on
  Bus Creator3 : BusCreator  Inputs=6  OutDataTypeStr=Bus: BoxParam3D  NonVirtualBus=on
  Bus Creator4 : BusCreator  Inputs=4  OutDataTypeStr=Bus: BoxParam2D  NonVirtualBus=on
  Bus Creator6 : BusCreator  Inputs=6  OutDataTypeStr=Bus: BoxParam3D  NonVirtualBus=on
  Bus Creator7 : BusCreator  Inputs=14  OutDataTypeStr=Bus: CameraMeasParam  NonVirtualBus=on
  Constant{1..3,9..12,16,18..30,35..39,43} (27 alike) : Constant  Value=single(0)
  Constant13 : Constant  Value=boolean(0)
  Constant14 : Constant  Value=uint8(2)
  Constant15 : Constant  Value=int16(-1)
  Constant17 : Constant  Value=single(10)
  Constant40 : Constant  Value=uint8(2)
  Constant41 : Constant  Value=single(zeros(4,4))
  Constant42 : Constant  Value=boolean(0)
  Constant44 : Constant  Value=single(10)
  Switch : Switch  Criteria=u2 ~= 0
  C2 : Outport
  wires:
  Bus Creator4/1 -> Bus Creator7/9  "Box2D"
  Bus Creator1/1 -> Bus Creator2/9  "Box2D"
  Bus Creator7/1 -> Switch/3
  Constant3/1 -> Bus Creator4/4  "Height"
  Constant44/1 -> Bus Creator7/13  "measConfidence"
  Constant19/1 -> Bus Creator3/2  "RefY"
  id/1 -> Bus Creator7/2, Bus Creator2/2, Switch/2  "measID"
  Bus Creator2/1 -> Switch/1
  Constant2/1 -> Bus Creator4/3  "Width"
  Constant12/1 -> Bus Creator1/4  "Height"
  Constant43/1 -> Bus Creator7/12  "ClassificationScore"
  Constant41/1 -> Bus Creator7/8  "NoiseCovarience"
  Constant20/1 -> Bus Creator3/3  "RefZ"
  Constant37/1 -> Bus Creator7/5  "py"
  Constant23/1 -> Bus Creator3/6  "LengthZ"
  Constant11/1 -> Bus Creator1/3  "Width"
  Constant18/1 -> Bus Creator3/1  "RefX"
  Constant9/1 -> Bus Creator1/1  "RefX"
  Constant27/1 -> Bus Creator6/4  "LengthX"
  Bus Creator3/1 -> Bus Creator2/10  "Box3D"
  Constant17/1 -> Bus Creator2/13  "measConfidence"
  py/1 -> Bus Creator2/5  "py"
  Constant36/1 -> Bus Creator7/4  "px"
  Constant16/1 -> Bus Creator2/12  "ClassificationScore"
  Constant42/1 -> Bus Creator7/14  "StationaryFlag"
  SensorData/1 -> Assignment/1
  px/1 -> Bus Creator2/4  "px"
  Constant39/1 -> Bus Creator7/7  "vy"
  Constant35/1 -> Bus Creator7/1  "TimeStamp"
  Constant38/1 -> Bus Creator7/6  "vx"
  TIME_STAMP/1 -> Bus Creator2/1  "TimeStamp"
  Switch/1 -> Assignment/2
  iter/1 -> Assignment/3
  Bus Creator6/1 -> Bus Creator7/10  "Box3D"
  Constant10/1 -> Bus Creator1/2  "RefY"
  NOISE_COV/1 -> Bus Creator2/8  "NoiseCovarience"
  Constant21/1 -> Bus Creator3/4  "LengthX"
  Constant1/1 -> Bus Creator4/2  "RefY"
  Constant25/1 -> Bus Creator6/2  "RefY"
  Constant26/1 -> Bus Creator6/3  "RefZ"
  Constant29/1 -> Bus Creator6/6  "LengthZ"
  Constant30/1 -> Bus Creator4/1  "RefX"
  vx/1 -> Bus Creator2/6  "vx"
  Constant13/1 -> Bus Creator2/14  "StationaryFlag"
  Constant22/1 -> Bus Creator3/5  "LengthY"
  Constant24/1 -> Bus Creator6/1  "RefX"
  Constant40/1 -> Bus Creator7/3  "cameraID"
  Constant28/1 -> Bus Creator6/5  "LengthY"
  Assignment/1 -> C2/1
  Constant15/1 -> Bus Creator7/11  "Classification"
  Constant14/1 -> Bus Creator2/3  "cameraID"
  vy/1 -> Bus Creator2/7  "vy"
  OBJ_TYPE/1 -> Bus Creator2/11  "Classification"

== system FusionMODEL_version1/SENSOR_MEASUREMENTS/RADAR_CAMERA_EGO_SENSOR_INTERFACE/CameraSensors/Camera3/ExtractMeasParam1 ==
  idx : Inport
  time : Inport  Port=2
  Constant : Constant  Value=CAM3_PX
  Constant1 : Constant  Value=CAM3_PY
  Constant2 : Constant  Value=CAM3_VX
  Constant3 : Constant  Value=CAM3_VY
  Constant4 : Constant  Value=CAM3_objClassID
  Constant5 : Constant  Value=CAM3_MeasNoise
  Constant6 : Constant  Value=CAM3_detTimeStamp
  Data Type Conversion : DataTypeConversion  OutDataTypeStr=int16
  MeasNoise : Selector  NumberOfDimensions=4  InputPortWidth=3  IndexOptions=Index vector (port),Select all,Select all,Index vector (port)  Indices=[1 3],1,1,1  OutputSizes=1,1,1,1
  PosX : Selector  NumberOfDimensions=2  InputPortWidth=3  IndexOptions=Index vector (port),Index vector (port)  Indices=[1 3],1  OutputSizes=1,1
  PosY : Selector  NumberOfDimensions=2  InputPortWidth=3  IndexOptions=Index vector (port),Index vector (port)  Indices=[1 3],1  OutputSizes=1,1
  Reshape : Reshape  OutputDimensionality=Customize  OutputDimensions=[4,4]
  VelX : Selector  NumberOfDimensions=2  InputPortWidth=3  IndexOptions=Index vector (port),Index vector (port)  Indices=[1 3],1  OutputSizes=1,1
  VelY : Selector  NumberOfDimensions=2  InputPortWidth=3  IndexOptions=Index vector (port),Index vector (port)  Indices=[1 3],1  OutputSizes=1,1
  snr : Selector  NumberOfDimensions=2  InputPortWidth=3  IndexOptions=Index vector (port),Index vector (port)  Indices=[1 3],1  OutputSizes=1,1
  timeStamp : Selector  NumberOfDimensions=2  InputPortWidth=3  IndexOptions=Select all,Index vector (port)  Indices=[1 3],1  OutputSizes=1,1
  PX : Outport
  PY : Outport  Port=2
  VX : Outport  Port=3
  VY : Outport  Port=4
  OBJ_TYPE : Outport  Port=5
  NOISE_COV : Outport  Port=6
  measCaptureTime : Outport  Port=7
  wires:
  Constant3/1 -> VelY/1
  Constant2/1 -> VelX/1
  VelY/1 -> VY/1
  Constant/1 -> PosX/1
  idx/1 -> MeasNoise/3, snr/3, VelY/3, VelX/3, PosY/3, PosX/3
  Constant1/1 -> PosY/1
  VelX/1 -> VX/1
  PosX/1 -> PX/1
  PosY/1 -> PY/1
  time/1 -> timeStamp/2, MeasNoise/2, snr/2, VelY/2, VelX/2, PosY/2, PosX/2
  Constant4/1 -> snr/1
  snr/1 -> Data Type Conversion/1
  Constant5/1 -> MeasNoise/1
  Constant6/1 -> timeStamp/1
  MeasNoise/1 -> Reshape/1
  timeStamp/1 -> measCaptureTime/1
  Reshape/1 -> NOISE_COV/1
  Data Type Conversion/1 -> OBJ_TYPE/1

== system FusionMODEL_version1/SENSOR_MEASUREMENTS/RADAR_CAMERA_EGO_SENSOR_INTERFACE/CameraSensors/Camera3/IsValid2 ==
  idx : Inport
  px : Inport  Port=2
  py : Inport  Port=3
  vx : Inport  Port=4
  vy : Inport  Port=5
  Abs{,1..3} (4 alike) : Abs
  Add : Sum  Inputs=++++
  Constant : Constant  Value=uint16(0)
  Data Type Conversion : DataTypeConversion  OutDataTypeStr=uint16
  Switch : Switch  Threshold=0.0001
  ID : Outport
  wires:
  Add/1 -> Switch/2
  Abs2/1 -> Add/3
  Constant/1 -> Switch/3
  Abs/1 -> Add/1
  px/1 -> Abs/1
  Abs3/1 -> Add/4
  Abs1/1 -> Add/2
  vy/1 -> Abs3/1
  py/1 -> Abs1/1
  vx/1 -> Abs2/1
  idx/1 -> Data Type Conversion/1
  Switch/1 -> ID/1
  Data Type Conversion/1 -> Switch/1

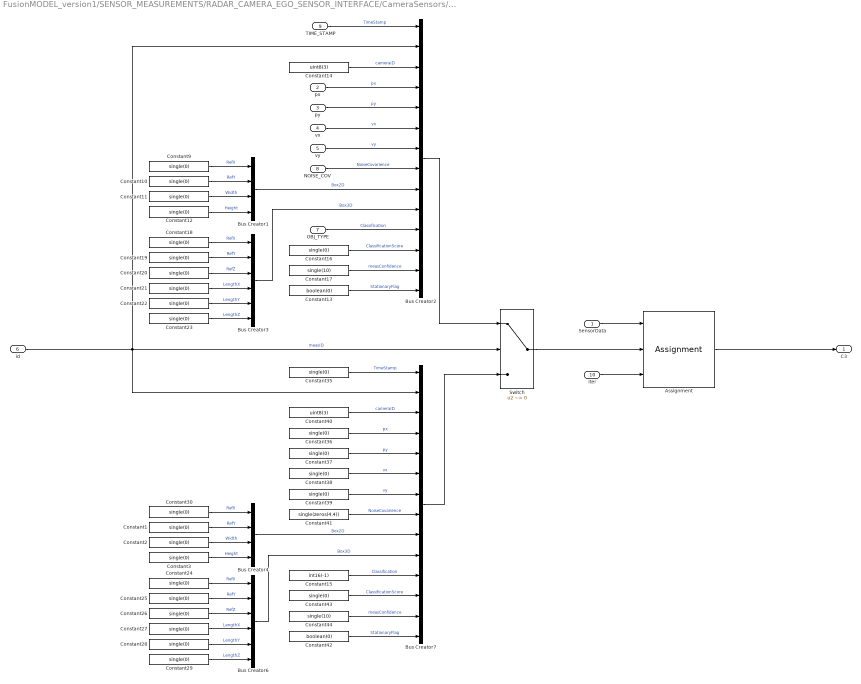
== system FusionMODEL_version1/SENSOR_MEASUREMENTS/RADAR_CAMERA_EGO_SENSOR_INTERFACE/CameraSensors/Camera3/Subsystem1 ==
  SensorData : Inport
  px : Inport  Port=2
  py : Inport  Port=3
  vx : Inport  Port=4
  vy : Inport  Port=5
  id : Inport  Port=6
  OBJ_TYPE : Inport  Port=7
  NOISE_COV : Inport  Port=8
  TIME_STAMP : Inport  Port=9
  iter : Inport  Port=10
  Assignment : Assignment  DiagnosticForDimensions=Warning  IndexOptions=Index vector (port)  Indices=1  OutputSizes=1
  Bus Creator1 : BusCreator  Inputs=4  OutDataTypeStr=Bus: BoxParam2D  NonVirtualBus=on
  Bus Creator2 : BusCreator  Inputs=14  OutDataTypeStr=Bus: CameraMeasParam  NonVirtualBus=on
  Bus Creator3 : BusCreator  Inputs=6  OutDataTypeStr=Bus: BoxParam3D  NonVirtualBus=on
  Bus Creator4 : BusCreator  Inputs=4  OutDataTypeStr=Bus: BoxParam2D  NonVirtualBus=on
  Bus Creator6 : BusCreator  Inputs=6  OutDataTypeStr=Bus: BoxParam3D  NonVirtualBus=on
  Bus Creator7 : BusCreator  Inputs=14  OutDataTypeStr=Bus: CameraMeasParam  NonVirtualBus=on
  Constant{1..3,9..12,16,18..30,35..39,43} (27 alike) : Constant  Value=single(0)
  Constant13 : Constant  Value=boolean(0)
  Constant14 : Constant  Value=uint8(3)
  Constant15 : Constant  Value=int16(-1)
  Constant17 : Constant  Value=single(10)
  Constant40 : Constant  Value=uint8(3)
  Constant41 : Constant  Value=single(zeros(4,4))
  Constant42 : Constant  Value=boolean(0)
  Constant44 : Constant  Value=single(10)
  Switch : Switch  Criteria=u2 ~= 0
  C3 : Outport
  wires:
  Bus Creator4/1 -> Bus Creator7/9  "Box2D"
  Bus Creator1/1 -> Bus Creator2/9  "Box2D"
  Bus Creator7/1 -> Switch/3
  Constant3/1 -> Bus Creator4/4  "Height"
  Constant44/1 -> Bus Creator7/13  "measConfidence"
  Constant19/1 -> Bus Creator3/2  "RefY"
  id/1 -> Bus Creator7/2, Bus Creator2/2, Switch/2  "measID"
  Bus Creator2/1 -> Switch/1
  Constant2/1 -> Bus Creator4/3  "Width"
  Constant12/1 -> Bus Creator1/4  "Height"
  Constant43/1 -> Bus Creator7/12  "ClassificationScore"
  Constant41/1 -> Bus Creator7/8  "NoiseCovarience"
  Constant20/1 -> Bus Creator3/3  "RefZ"
  Constant37/1 -> Bus Creator7/5  "py"
  Constant23/1 -> Bus Creator3/6  "LengthZ"
  Constant11/1 -> Bus Creator1/3  "Width"
  Constant18/1 -> Bus Creator3/1  "RefX"
  Constant9/1 -> Bus Creator1/1  "RefX"
  Constant27/1 -> Bus Creator6/4  "LengthX"
  Bus Creator3/1 -> Bus Creator2/10  "Box3D"
  Constant17/1 -> Bus Creator2/13  "measConfidence"
  py/1 -> Bus Creator2/5  "py"
  Constant36/1 -> Bus Creator7/4  "px"
  Constant16/1 -> Bus Creator2/12  "ClassificationScore"
  Constant42/1 -> Bus Creator7/14  "StationaryFlag"
  SensorData/1 -> Assignment/1
  px/1 -> Bus Creator2/4  "px"
  Constant39/1 -> Bus Creator7/7  "vy"
  Constant35/1 -> Bus Creator7/1  "TimeStamp"
  Constant38/1 -> Bus Creator7/6  "vx"
  TIME_STAMP/1 -> Bus Creator2/1  "TimeStamp"
  Switch/1 -> Assignment/2
  iter/1 -> Assignment/3
  Bus Creator6/1 -> Bus Creator7/10  "Box3D"
  Constant10/1 -> Bus Creator1/2  "RefY"
  NOISE_COV/1 -> Bus Creator2/8  "NoiseCovarience"
  Constant21/1 -> Bus Creator3/4  "LengthX"
  Constant1/1 -> Bus Creator4/2  "RefY"
  Constant25/1 -> Bus Creator6/2  "RefY"
  Constant26/1 -> Bus Creator6/3  "RefZ"
  Constant29/1 -> Bus Creator6/6  "LengthZ"
  Constant30/1 -> Bus Creator4/1  "RefX"
  vx/1 -> Bus Creator2/6  "vx"
  Constant13/1 -> Bus Creator2/14  "StationaryFlag"
  Constant22/1 -> Bus Creator3/5  "LengthY"
  Constant24/1 -> Bus Creator6/1  "RefX"
  Constant40/1 -> Bus Creator7/3  "cameraID"
  Constant28/1 -> Bus Creator6/5  "LengthY"
  Assignment/1 -> C3/1
  Constant15/1 -> Bus Creator7/11  "Classification"
  Constant14/1 -> Bus Creator2/3  "cameraID"
  vy/1 -> Bus Creator2/7  "vy"
  OBJ_TYPE/1 -> Bus Creator2/11  "Classification"

== system FusionMODEL_version1/SENSOR_MEASUREMENTS/RADAR_CAMERA_EGO_SENSOR_INTERFACE/CameraSensors/Camera4/ExtractMeasParam1 ==
  idx : Inport
  time : Inport  Port=2
  Constant : Constant  Value=CAM4_PX
  Constant1 : Constant  Value=CAM4_PY
  Constant2 : Constant  Value=CAM4_VX
  Constant3 : Constant  Value=CAM4_VY
  Constant4 : Constant  Value=CAM4_objClassID
  Constant5 : Constant  Value=CAM4_MeasNoise
  Constant6 : Constant  Value=CAM4_detTimeStamp
  Data Type Conversion : DataTypeConversion  OutDataTypeStr=int16
  MeasNoise : Selector  NumberOfDimensions=4  InputPortWidth=3  IndexOptions=Index vector (port),Select all,Select all,Index vector (port)  Indices=[1 3],1,1,1  OutputSizes=1,1,1,1
  PosX : Selector  NumberOfDimensions=2  InputPortWidth=3  IndexOptions=Index vector (port),Index vector (port)  Indices=[1 3],1  OutputSizes=1,1
  PosY : Selector  NumberOfDimensions=2  InputPortWidth=3  IndexOptions=Index vector (port),Index vector (port)  Indices=[1 3],1  OutputSizes=1,1
  Reshape : Reshape  OutputDimensionality=Customize  OutputDimensions=[4,4]
  VelX : Selector  NumberOfDimensions=2  InputPortWidth=3  IndexOptions=Index vector (port),Index vector (port)  Indices=[1 3],1  OutputSizes=1,1
  VelY : Selector  NumberOfDimensions=2  InputPortWidth=3  IndexOptions=Index vector (port),Index vector (port)  Indices=[1 3],1  OutputSizes=1,1
  snr : Selector  NumberOfDimensions=2  InputPortWidth=3  IndexOptions=Index vector (port),Index vector (port)  Indices=[1 3],1  OutputSizes=1,1
  timeStamp : Selector  NumberOfDimensions=2  InputPortWidth=3  IndexOptions=Select all,Index vector (port)  Indices=[1 3],1  OutputSizes=1,1
  PX : Outport
  PY : Outport  Port=2
  VX : Outport  Port=3
  VY : Outport  Port=4
  OBJ_TYPE : Outport  Port=5
  NOISE_COV : Outport  Port=6
  measCaptureTime : Outport  Port=7
  wires:
  Constant3/1 -> VelY/1
  Constant2/1 -> VelX/1
  VelY/1 -> VY/1
  Constant/1 -> PosX/1
  idx/1 -> MeasNoise/3, snr/3, VelY/3, VelX/3, PosY/3, PosX/3
  Constant1/1 -> PosY/1
  VelX/1 -> VX/1
  PosX/1 -> PX/1
  PosY/1 -> PY/1
  time/1 -> timeStamp/2, MeasNoise/2, snr/2, VelY/2, VelX/2, PosY/2, PosX/2
  Constant4/1 -> snr/1
  snr/1 -> Data Type Conversion/1
  Constant5/1 -> MeasNoise/1
  Constant6/1 -> timeStamp/1
  MeasNoise/1 -> Reshape/1
  timeStamp/1 -> measCaptureTime/1
  Reshape/1 -> NOISE_COV/1
  Data Type Conversion/1 -> OBJ_TYPE/1

== system FusionMODEL_version1/SENSOR_MEASUREMENTS/RADAR_CAMERA_EGO_SENSOR_INTERFACE/CameraSensors/Camera4/IsValid2 ==
  idx : Inport
  px : Inport  Port=2
  py : Inport  Port=3
  vx : Inport  Port=4
  vy : Inport  Port=5
  Abs{,1..3} (4 alike) : Abs
  Add : Sum  Inputs=++++
  Constant : Constant  Value=uint16(0)
  Data Type Conversion : DataTypeConversion  OutDataTypeStr=uint16
  Switch : Switch  Threshold=0.0001
  ID : Outport
  wires:
  Add/1 -> Switch/2
  Abs2/1 -> Add/3
  Constant/1 -> Switch/3
  Abs/1 -> Add/1
  px/1 -> Abs/1
  Abs3/1 -> Add/4
  Abs1/1 -> Add/2
  vy/1 -> Abs3/1
  py/1 -> Abs1/1
  vx/1 -> Abs2/1
  idx/1 -> Data Type Conversion/1
  Switch/1 -> ID/1
  Data Type Conversion/1 -> Switch/1
